simulink model "new_control"  (R2024b)
settings: Solver=FixedStepAuto  StartTime=0.0  StopTime=inf  FixedStep=0.01  RelTol=1e-3  EnableMultiTasking=on
undefined symbols (not defined in the file or in its folder): Discrete, qbreak, Time
libraries: simulink x70, arduinolib x30, dspswit3 x13, arduinosensorlib x2, ctrlSharedLib x2
(part 2 of 4)

== system new_control/Initialize Function/Config_R/Enter Config Mode ==
  Compare To Zero8 : simulink/Logic and Bit Operations/Compare To Zero  relop===  OutDataTypeStr=boolean
  Constant5 : Constant  Value=0x00
  Start_Config_R : arduinolib/I2C Write  I2CModule=0  Mode=Master  SlaveAddress=0x29  SlaveByteOrder=BigEndian  Direction=Transmitter  RegisterAddressMode=on  RegisterAddress=0x3D  SlaveDataType=uint8  DataLength=1  NoAck=off  RepeatedStart=off  OutputStatus=on  blockPlatform=ARDUINO
  Status : Outport
  wires:
  Start_Config_R/1 -> Compare To Zero8/1  "0 for success"
  Constant5/1 -> Start_Config_R/1
  Compare To Zero8/1 -> Status/1

== system new_control/Initialize Function/Config_R/Start Fused (NDOF) Mode ==
  Enable : EnablePort
  Compare To Constant1 : simulink/Logic and Bit Operations/Compare To Constant  relop===  const=0  OutDataTypeStr=boolean
  Constant4 : Constant  Value=0x0C
  I2C Write8 : arduinolib/I2C Write  I2CModule=0  Mode=Master  SlaveAddress=0x29  SlaveByteOrder=BigEndian  Direction=Transmitter  RegisterAddressMode=on  RegisterAddress=0x3D  SlaveDataType=uint8  DataLength=1  NoAck=off  RepeatedStart=off  OutputStatus=on  blockPlatform=ARDUINO
  Status : Outport
  wires:
  Compare To Constant1/1 -> Status/1
  Constant4/1 -> I2C Write8/1
  I2C Write8/1 -> Compare To Constant1/1  "0: success"

== system new_control/Initialize Function/Config_R/X=Z, Y=Y, Z=X ==
  Enable : EnablePort
  Compare To Constant : simulink/Logic and Bit Operations/Compare To Constant  relop=~=  const=hex2dec('06')  OutDataTypeStr=boolean
  Compare To Constant1 : simulink/Logic and Bit Operations/Compare To Constant  relop===  const=hex2dec('06')  OutDataTypeStr=boolean
  Enabled Subsystem : Subsystem  TreatAsAtomicUnit=on
  I2C Read : arduinolib/I2C Read  I2CModule=0  Mode=Master  SlaveAddress=0x29  SlaveByteOrder=LittleEndian  Direction=Receiver  RegisterAddressMode=on  RegisterAddress=0x41  SlaveDataType=uint8  DataLength=1  NoAck=off  RepeatedStart=off  OutputStatus=off  blockPlatform=ARDUINO  SampleTime=-1
  OR : Logic  Operator=OR  IconShape=distinctive  AllPortsSameDT=off  OutDataTypeStr=boolean
  Status : Outport
  wires:
  I2C Read/1 -> Compare To Constant1/1, Compare To Constant/1
  Compare To Constant1/1 -> OR/2
  Compare To Constant/1 -> Enabled Subsystem/Enable
  Enabled Subsystem/1(Status) -> OR/1
  OR/1 -> Status/1

== system new_control/Initialize Function/Config_R/Z = -Z ==
  note: 0x01: Z = -Z
  Enable : EnablePort
  Compare To Constant : simulink/Logic and Bit Operations/Compare To Constant  relop=~=  const=hex2dec('01')  OutDataTypeStr=boolean
  Compare To Constant1 : simulink/Logic and Bit Operations/Compare To Constant  relop===  const=hex2dec('01')  OutDataTypeStr=boolean
  OR : Logic  Operator=OR  IconShape=distinctive  AllPortsSameDT=off  OutDataTypeStr=boolean
  Read : arduinolib/I2C Read  I2CModule=0  Mode=Master  SlaveAddress=0x29  SlaveByteOrder=LittleEndian  Direction=Receiver  RegisterAddressMode=on  RegisterAddress=0x42  SlaveDataType=uint8  DataLength=1  NoAck=off  RepeatedStart=off  OutputStatus=off  blockPlatform=ARDUINO  SampleTime=-1
  Write : Subsystem  TreatAsAtomicUnit=on
  Status : Outport
  wires:
  Write/1(Status) -> OR/1
  Compare To Constant/1 -> Write/Enable
  Read/1 -> Compare To Constant1/1, Compare To Constant/1
  Compare To Constant1/1 -> OR/2
  OR/1 -> Status/1

== system new_control/LEFT LEG/GAIT PHASE BLOCK/CENTERING AND NORMALIZING ==
  Angle max : Inport
  Angle min : Inport  Port=2
  Vel max : Inport  Port=3
  Vel min : Inport  Port=4
  Trigger : TriggerPort  VariantControl=(inherit)  PortDimensions=1
  Abs : Abs  SaturateOnIntegerOverflow=off
  Abs1 : Abs  SaturateOnIntegerOverflow=off
  Constant : Constant  Value=0.5
  Constant1 : Constant  Value=0.5
  Divide : Product  Inputs=/*
  Product : Product
  Product1 : Product
  Sum : Sum
  Sum1 : Sum
  Sum2 : Sum  Inputs=+-
  Sum3 : Sum  Inputs=+-
  Switch : Switch  Criteria=u2 > Threshold  SaturateOnIntegerOverflow=off  InputSameDT=off
  Center vel : Outport
  Center angle : Outport  Port=2
  Gamma : Outport  Port=3
  wires:
  Angle max/1 -> Sum2/1, Sum/1
  Angle min/1 -> Sum2/2, Sum/2
  Sum/1 -> Product/1
  Constant/1 -> Product/2
  Product/1 -> Center angle/1
  Constant1/1 -> Product1/2
  Sum1/1 -> Product1/1
  Vel max/1 -> Sum3/1, Sum1/1
  Vel min/1 -> Sum3/2, Sum1/2
  Product1/1 -> Center vel/1
  Sum2/1 -> Abs/1
  Sum3/1 -> Abs1/1
  Abs/1 -> Switch/2, Switch/1
  Switch/1 -> Divide/1
  Abs1/1 -> Divide/2, Switch/3
  Divide/1 -> Gamma/1

== system new_control/LEFT LEG/GAIT PHASE BLOCK/LOGIC FOR THE BEGINNING ==
  Enable : EnablePort
  Constant : Constant  Value=0
  Phase to zero : Outport
  wires:
  Constant/1 -> Phase to zero/1

== system new_control/LEFT LEG/GAIT PHASE BLOCK/STRIDE EVENT DETECTOR ==
  In1 : Inport
  angle : Inport  Port=2
  Enable : EnablePort
  AND : Logic  IconShape=distinctive  AllPortsSameDT=off  OutDataTypeStr=boolean
  Hit Crossing5 : HitCross  HitCrossingOffset=-0.1  HitCrossingDirection=falling
  Relational Operator : RelationalOperator  OutDataTypeStr=boolean  RndMeth=Simplest  InputSameDT=off
  ~5 degrees : Constant  Value=0.08
  Out1 : Outport
  wires:
  In1/1 -> Hit Crossing5/1
  angle/1 -> Relational Operator/1
  Relational Operator/1 -> AND/2
  ~5 degrees/1 -> Relational Operator/2
  Hit Crossing5/1 -> Out1/1

== system new_control/LEFT LEG/GAIT PHASE BLOCK/Subsystem ==
  Input : Inport
  Trigger : TriggerPort  VariantControl=Variant  PortDimensions=1
  Angle min : Outport
  wires:
  Input/1 -> Angle min/1

== system new_control/LEFT LEG/GAIT PHASE BLOCK/Subsystem2 ==
  Input : Inport
  Trigger : TriggerPort  VariantControl=Variant  PortDimensions=1
  Angle max : Outport
  wires:
  Input/1 -> Angle max/1

== system new_control/LEFT LEG/GAIT PHASE BLOCK/Subsystem4 ==
  Input : Inport
  Trigger : TriggerPort  VariantControl=Variant  PortDimensions=1
  Vel min : Outport
  wires:
  Input/1 -> Vel min/1

== system new_control/LEFT LEG/GAIT PHASE BLOCK/Subsystem5 ==
  Input : Inport
  Trigger : TriggerPort  VariantControl=Variant  PortDimensions=1
  Vel max : Outport
  wires:
  Input/1 -> Vel max/1

== system new_control/LEFT LEG/Subsystem/SIGMOID SCALING ==
  note: a^n / (a^n + 1)
      |
      | The higher n, the more low amplitudes are scaled down
  PORTRAIT RADIUS : Inport
  Sigmoid Power : Inport  Port=2
  Constant2 : Constant
  Divide : Product  Inputs=*/
  Power : Math  Operator=pow
  Scale to 1 : Saturate  UpperLimit=1  LowerLimit=0
  Sum1 : Sum
  Out1 : Outport
  wires:
  Sum1/1 -> Divide/2
  Sigmoid Power/1 -> Power/2  "sig_power_L"
  Constant2/1 -> Sum1/2
  Scale to 1/1 -> Out1/1
  Power/1 -> Divide/1, Sum1/1
  PORTRAIT RADIUS/1 -> Power/1
  Divide/1 -> Scale to 1/1

== system new_control/RIGHT LEG/GAIT PHASE BLOCK/CENTERING AND NORMALIZING ==
  Angle max : Inport
  Angle min : Inport  Port=2
  Vel max : Inport  Port=3
  Vel min : Inport  Port=4
  Trigger : TriggerPort  VariantControl=(inherit)  PortDimensions=1
  Abs : Abs  SaturateOnIntegerOverflow=off
  Abs1 : Abs  SaturateOnIntegerOverflow=off
  Constant : Constant  Value=0.5
  Constant1 : Constant  Value=0.5
  Divide : Product  Inputs=/*
  Product : Product
  Product1 : Product
  Sum : Sum
  Sum1 : Sum
  Sum2 : Sum  Inputs=+-
  Sum3 : Sum  Inputs=+-
  Switch : Switch  Criteria=u2 > Threshold  SaturateOnIntegerOverflow=off  InputSameDT=off
  Center vel : Outport
  Center angle : Outport  Port=2
  Gamma : Outport  Port=3
  wires:
  Angle max/1 -> Sum2/1, Sum/1
  Angle min/1 -> Sum2/2, Sum/2
  Sum/1 -> Product/1
  Constant/1 -> Product/2
  Product/1 -> Center angle/1
  Constant1/1 -> Product1/2
  Sum1/1 -> Product1/1
  Vel max/1 -> Sum3/1, Sum1/1
  Vel min/1 -> Sum3/2, Sum1/2
  Product1/1 -> Center vel/1
  Sum2/1 -> Abs/1
  Sum3/1 -> Abs1/1
  Abs/1 -> Switch/2, Switch/1
  Switch/1 -> Divide/1
  Abs1/1 -> Divide/2, Switch/3
  Divide/1 -> Gamma/1

== system new_control/RIGHT LEG/GAIT PHASE BLOCK/LOGIC FOR THE BEGINNING ==
  Enable : EnablePort
  Constant : Constant  Value=0
  Phase to zero : Outport
  wires:
  Constant/1 -> Phase to zero/1

== system new_control/RIGHT LEG/GAIT PHASE BLOCK/STRIDE EVENT DETECTOR ==
  In1 : Inport
  angle : Inport  Port=2
  Enable : EnablePort
  AND : Logic  IconShape=distinctive  AllPortsSameDT=off  OutDataTypeStr=boolean
  Hit Crossing5 : HitCross  HitCrossingOffset=-0.1  HitCrossingDirection=falling
  Relational Operator : RelationalOperator  OutDataTypeStr=boolean  RndMeth=Simplest  InputSameDT=off
  ~5 degrees : Constant  Value=0.08
  Out1 : Outport
  wires:
  In1/1 -> Hit Crossing5/1
  angle/1 -> Relational Operator/1
  Relational Operator/1 -> AND/2
  ~5 degrees/1 -> Relational Operator/2
  Hit Crossing5/1 -> Out1/1

== system new_control/RIGHT LEG/GAIT PHASE BLOCK/Subsystem ==
  Input : Inport
  Trigger : TriggerPort  VariantControl=Variant  PortDimensions=1
  Angle min : Outport
  wires:
  Input/1 -> Angle min/1

== system new_control/RIGHT LEG/GAIT PHASE BLOCK/Subsystem2 ==
  Input : Inport
  Trigger : TriggerPort  VariantControl=Variant  PortDimensions=1
  Angle max : Outport
  wires:
  Input/1 -> Angle max/1

== system new_control/RIGHT LEG/GAIT PHASE BLOCK/Subsystem4 ==
  Input : Inport
  Trigger : TriggerPort  VariantControl=Variant  PortDimensions=1
  Vel min : Outport
  wires:
  Input/1 -> Vel min/1

== system new_control/RIGHT LEG/GAIT PHASE BLOCK/Subsystem5 ==
  Input : Inport
  Trigger : TriggerPort  VariantControl=Variant  PortDimensions=1
  Vel max : Outport
  wires:
  Input/1 -> Vel max/1

== system new_control/RIGHT LEG/Subsystem/SIGMOID SCALING ==
  note: a^n / (a^n + 1)
      |
      | The higher n, the more low amplitudes are scaled down
  PORTRAIT RADIUS : Inport
  sigmoid_power : Inport  Port=2
  Constant2 : Constant
  Divide : Product  Inputs=*/
  Power : Math  Operator=pow
  Scale to 1 : Saturate  UpperLimit=1  LowerLimit=0
  Sum1 : Sum
  Out1 : Outport
  wires:
  Sum1/1 -> Divide/2
  sigmoid_power/1 -> Power/2
  Constant2/1 -> Sum1/2
  Scale to 1/1 -> Out1/1
  Power/1 -> Divide/1, Sum1/1
  PORTRAIT RADIUS/1 -> Power/1
  Divide/1 -> Scale to 1/1

== system new_control/Subsystem1/Left Motor Velocity1/Motor Actual Position Receive ==
  SWITCH : Inport
  Bus Selector1 : BusSelector  OutputSignals=Data
  CAN Receive : arduinolib/CAN Receive  outputDataType=CAN Msg  identifierType=Standard (11-bit identifier)  messageId=0  msgLength=8  SampleTime=0.01  outputError=off  outputRemote=off
  CHINESE CORRECTION : Subsystem
  Constant1 : Constant  Value=0
  Constant3 : Constant
  Data Type Conversion2 : DataTypeConversion  OutDataTypeStr=uint16  SaturateOnIntegerOverflow=off  RndMeth=Floor
  Delay : Delay  DelayLength=1
  Delay2 : Delay
  Memory2 : Memory
  N-Sample Switch2 : dspswit3/N-Sample Switch  N=10  reset=on  TriggerType=Rising edge  Ts=0.01
  Sum : Sum  Inputs=-|+
  Switch2 : Switch  Criteria=u2 > Threshold  SaturateOnIntegerOverflow=off  InputSameDT=off
  Terminator1 : Terminator
  Unpack2 : Subsystem
  MOTOR POSITION : Outport
  MOTOR SPEED : Outport  Port=2
  MOTOR TORQUE : Outport  Port=3
  wires:
  Switch2/1 -> Sum/1, Delay2/1
  CAN Receive/1 -> Bus Selector1/1
  SWITCH/1 -> N-Sample Switch2/3, CHINESE CORRECTION/Enable
  N-Sample Switch2/1 -> Switch2/2
  Memory2/1 -> Switch2/1
  Constant1/1 -> N-Sample Switch2/1
  Sum/1 -> Delay/1
  Unpack2/2(speed) -> MOTOR SPEED/1  "MOTOR SPEED"
  Delay2/1 -> Memory2/1
  Bus Selector1/1 -> Data Type Conversion2/1  "<Data>"
  CHINESE CORRECTION/1(Out1) -> Sum/2, Switch2/3
  Constant3/1 -> N-Sample Switch2/2
  Unpack2/1(position) -> CHINESE CORRECTION/1(position)  "MOTOR POS"
  Data Type Conversion2/1 -> Unpack2/1(Data)
  CAN Receive/2 -> Terminator1/1
  Delay/1 -> MOTOR POSITION/1
  Unpack2/3(torque) -> MOTOR TORQUE/1  "MOTOR TORQUE"

== system new_control/Subsystem1/Left Motor Velocity1/Subsystem ==
  Motor command : Inport
  SWITCH : Inport  Port=2
  CAN Pack1 : Subsystem
  CAN Transmit1 : arduinolib/CAN Transmit  inputDataType=Raw data  BlockingMode_=on  BlockTimeout_=1  outputStatus=off  identifierType=Standard (11-bit identifier)  messageId=4  msgLength=8  remoteFrame=off
  Constant7 : Constant  Value=0  OutDataTypeStr=single  SampleTime=0.01
  DISABLE1 : Constant  Value=269.7/18  OutDataTypeStr=single
  Data Type Conversion3 : DataTypeConversion  OutDataTypeStr=single  SaturateOnIntegerOverflow=off  RndMeth=Floor
  Demux1 : Demux  Outputs=5
  ENABLE1 : Constant  Value=14.975  OutDataTypeStr=single
  IsNaN : RelationalOperator  Operator=isNaN  OutDataTypeStr=boolean  RndMeth=Simplest  InputSameDT=off
  N-Sample Switch4 : dspswit3/N-Sample Switch  N=15  reset=on  TriggerType=Either edge  Ts=0.01
  Rate Transition : RateTransition  OutPortSampleTime=0.01
  Subsystem2 : Subsystem
  Switch : Switch  Criteria=u2 > Threshold  SaturateOnIntegerOverflow=off  InputSameDT=off
  Switch3 : Switch  Criteria=u2 > Threshold  SaturateOnIntegerOverflow=off  InputSameDT=off
  wires:
  Demux1/4 -> CAN Pack1/4(Kd)
  Data Type Conversion3/1 -> Subsystem2/2(Velocity)
  Switch3/1 -> Subsystem2/1(Enable)
  Demux1/1 -> CAN Pack1/1(Position)
  Motor command/1 -> Data Type Conversion3/1, IsNaN/1
  Demux1/5 -> CAN Pack1/5(Torque)
  ENABLE1/1 -> Switch3/1
  Demux1/2 -> CAN Pack1/2(Velocity)
  Rate Transition/1 -> N-Sample Switch4/3
  IsNaN/1 -> Switch/2
  DISABLE1/1 -> Switch3/3
  Subsystem2/1(Enter_motor_mode) -> N-Sample Switch4/1
  Demux1/3 -> CAN Pack1/3(Kp)
  N-Sample Switch4/1 -> Demux1/1
  Switch/1 -> Rate Transition/1, Switch3/2
  CAN Pack1/1(CAN Data) -> CAN Transmit1/1
  Subsystem2/2(Velocity_value) -> N-Sample Switch4/2
  Constant7/1 -> Switch/1
  SWITCH/1 -> Switch/3

== system new_control/Subsystem1/PID1/Subsystem2 ==
  x : Inport
  Constant : Constant  Value=2
  Integrator1 : Integrator  InitialConditionSource=external
  Integrator2 : Integrator
  Product : Product  RndMeth=Zero
  Product1 : Product  RndMeth=Zero
  Product2 : Product  Inputs=3  RndMeth=Zero
  Sum : Sum  Inputs=|+-
  Sum1 : Sum  Inputs=|+-
  wn : Constant  Value=wn
  x0 : Constant  Value=x0
  zt : Constant  Value=zt
  y : Outport  VectorParamsAs1DForOutWhenUnconnected=off
  yd : Outport  Port=2  VectorParamsAs1DForOutWhenUnconnected=off
  wires:
  Sum/1 -> Product/2
  wn/1 -> Product/1, Product1/1
  Sum1/1 -> Sum/1
  x0/1 -> Integrator1/2
  Integrator2/1 -> Product1/2, Product2/1
  Product/1 -> Integrator2/1
  x/1 -> Sum1/1
  Product1/1 -> Integrator1/1, yd/1
  Integrator1/1 -> Sum1/2, y/1
  Product2/1 -> Sum/2
  zt/1 -> Product2/3
  Constant/1 -> Product2/2

== system new_control/Subsystem1/PID2/Subsystem2 ==
  x : Inport
  Constant : Constant  Value=2
  Integrator1 : Integrator  InitialConditionSource=external
  Integrator2 : Integrator
  Product : Product  RndMeth=Zero
  Product1 : Product  RndMeth=Zero
  Product2 : Product  Inputs=3  RndMeth=Zero
  Sum : Sum  Inputs=|+-
  Sum1 : Sum  Inputs=|+-
  wn : Constant  Value=wn
  x0 : Constant  Value=x0
  zt : Constant  Value=zt
  y : Outport  VectorParamsAs1DForOutWhenUnconnected=off
  yd : Outport  Port=2  VectorParamsAs1DForOutWhenUnconnected=off
  wires:
  Sum/1 -> Product/2
  wn/1 -> Product/1, Product1/1
  Sum1/1 -> Sum/1
  x0/1 -> Integrator1/2
  Integrator2/1 -> Product1/2, Product2/1
  Product/1 -> Integrator2/1
  x/1 -> Sum1/1
  Product1/1 -> Integrator1/1, yd/1
  Integrator1/1 -> Sum1/2, y/1
  Product2/1 -> Sum/2
  zt/1 -> Product2/3
  Constant/1 -> Product2/2

== system new_control/Subsystem1/Right Motor Velocity1/Motor Actual Position Receive ==
  SWITCH : Inport
  Bus Selector1 : BusSelector  OutputSignals=Data
  CAN Receive : arduinolib/CAN Receive  outputDataType=CAN Msg  identifierType=Standard (11-bit identifier)  messageId=0  msgLength=8  SampleTime=0.01  outputError=off  outputRemote=off
  CHINESE CORRECTION : Subsystem
  Constant1 : Constant  Value=0
  Constant3 : Constant
  Data Type Conversion2 : DataTypeConversion  OutDataTypeStr=uint16  SaturateOnIntegerOverflow=off  RndMeth=Floor
  Delay : Delay  DelayLength=1
  Delay2 : Delay
  Memory2 : Memory
  N-Sample Switch2 : dspswit3/N-Sample Switch  N=10  reset=on  TriggerType=Rising edge  Ts=0.01
  Sum : Sum  Inputs=-|+
  Switch2 : Switch  Criteria=u2 > Threshold  SaturateOnIntegerOverflow=off  InputSameDT=off
  Terminator1 : Terminator
  Unpack2 : Subsystem
  MOTOR POSITION : Outport
  MOTOR SPEED : Outport  Port=2
  MOTOR TORQUE : Outport  Port=3
  wires:
  Switch2/1 -> Sum/1, Delay2/1
  CAN Receive/1 -> Bus Selector1/1
  SWITCH/1 -> N-Sample Switch2/3, CHINESE CORRECTION/Enable
  N-Sample Switch2/1 -> Switch2/2
  Memory2/1 -> Switch2/1
  Constant1/1 -> N-Sample Switch2/1
  Sum/1 -> Delay/1
  Unpack2/2(speed) -> MOTOR SPEED/1  "MOTOR SPEED"
  Delay2/1 -> Memory2/1
  Bus Selector1/1 -> Data Type Conversion2/1  "<Data>"
  CHINESE CORRECTION/1(Out1) -> Sum/2, Switch2/3
  Constant3/1 -> N-Sample Switch2/2
  Unpack2/1(position) -> CHINESE CORRECTION/1(position)  "MOTOR POS"
  Data Type Conversion2/1 -> Unpack2/1(Data)
  CAN Receive/2 -> Terminator1/1
  Delay/1 -> MOTOR POSITION/1
  Unpack2/3(torque) -> MOTOR TORQUE/1  "MOTOR TORQUE"

== system new_control/Subsystem1/Right Motor Velocity1/Subsystem ==
  Motor command : Inport
  SWITCH : Inport  Port=2
  CAN Pack1 : Subsystem
  CAN Transmit1 : arduinolib/CAN Transmit  inputDataType=Raw data  BlockingMode_=on  BlockTimeout_=1  outputStatus=off  identifierType=Standard (11-bit identifier)  messageId=3  msgLength=8  remoteFrame=off
  Constant7 : Constant  Value=0  OutDataTypeStr=single  SampleTime=0.01
  DISABLE1 : Constant  Value=269.7/18  OutDataTypeStr=single
  Data Type Conversion3 : DataTypeConversion  OutDataTypeStr=single  SaturateOnIntegerOverflow=off  RndMeth=Floor
  Demux1 : Demux  Outputs=5
  ENABLE1 : Constant  Value=14.975  OutDataTypeStr=single
  IsNaN : RelationalOperator  Operator=isNaN  OutDataTypeStr=boolean  RndMeth=Simplest  InputSameDT=off
  N-Sample Switch4 : dspswit3/N-Sample Switch  N=15  reset=on  TriggerType=Either edge  Ts=0.01
  Rate Transition : RateTransition  OutPortSampleTime=0.01
  Subsystem2 : Subsystem
  Switch : Switch  Criteria=u2 > Threshold  SaturateOnIntegerOverflow=off  InputSameDT=off
  Switch3 : Switch  Criteria=u2 > Threshold  SaturateOnIntegerOverflow=off  InputSameDT=off
  wires:
  Demux1/4 -> CAN Pack1/4(Kd)
  Data Type Conversion3/1 -> Subsystem2/2(Velocity)
  Switch3/1 -> Subsystem2/1(Enable)
  Demux1/1 -> CAN Pack1/1(Position)
  Motor command/1 -> Data Type Conversion3/1, IsNaN/1
  Demux1/5 -> CAN Pack1/5(Torque)
  ENABLE1/1 -> Switch3/1
  Demux1/2 -> CAN Pack1/2(Velocity)
  Rate Transition/1 -> N-Sample Switch4/3
  IsNaN/1 -> Switch/2
  DISABLE1/1 -> Switch3/3
  Subsystem2/1(Enter_motor_mode) -> N-Sample Switch4/1
  Demux1/3 -> CAN Pack1/3(Kp)
  N-Sample Switch4/1 -> Demux1/1
  Switch/1 -> Rate Transition/1, Switch3/2
  CAN Pack1/1(CAN Data) -> CAN Transmit1/1
  Subsystem2/2(Velocity_value) -> N-Sample Switch4/2
  Constant7/1 -> Switch/1
  SWITCH/1 -> Switch/3

== system new_control/Subsystem3/Left Motor Velocity/Motor Actual Position Receive ==
  SWITCH : Inport
  Bus Selector1 : BusSelector  OutputSignals=Data
  CAN Receive : arduinolib/CAN Receive  Priority=4  outputDataType=CAN Msg  identifierType=Standard (11-bit identifier)  messageId=0  msgLength=8  SampleTime=0.01  outputError=off  outputRemote=off
  CHINESE CORRECTION : Subsystem
  Constant1 : Constant  Value=0
  Constant3 : Constant
  Data Type Conversion2 : DataTypeConversion  OutDataTypeStr=uint16  SaturateOnIntegerOverflow=off  RndMeth=Floor
  Delay : Delay  DelayLength=1
  Delay2 : Delay
  Memory2 : Memory
  N-Sample Switch2 : dspswit3/N-Sample Switch  N=10  reset=on  TriggerType=Rising edge  Ts=0.01
  Sum : Sum  Inputs=-|+
  Switch2 : Switch  Criteria=u2 > Threshold  SaturateOnIntegerOverflow=off  InputSameDT=off
  Terminator1 : Terminator
  Unpack2 : Subsystem
  Zero-Order Hold1 : ZeroOrderHold  SampleTime=0.01
  MOTOR POSITION : Outport
  MOTOR SPEED : Outport  Port=2
  MOTOR TORQUE : Outport  Port=3
  wires:
  Switch2/1 -> Sum/1, Delay2/1
  CAN Receive/1 -> Bus Selector1/1
  SWITCH/1 -> Zero-Order Hold1/1
  N-Sample Switch2/1 -> Switch2/2
  Memory2/1 -> Switch2/1
  Constant1/1 -> N-Sample Switch2/1
  Sum/1 -> Delay/1
  Unpack2/2(speed) -> MOTOR SPEED/1  "MOTOR SPEED"
  Delay2/1 -> Memory2/1
  Bus Selector1/1 -> Data Type Conversion2/1  "<Data>"
  CHINESE CORRECTION/1(Out1) -> Sum/2, Switch2/3
  Constant3/1 -> N-Sample Switch2/2
  Unpack2/1(position) -> CHINESE CORRECTION/1(position)  "MOTOR POS"
  Data Type Conversion2/1 -> Unpack2/1(Data)
  CAN Receive/2 -> Terminator1/1
  Delay/1 -> MOTOR POSITION/1
  Unpack2/3(torque) -> MOTOR TORQUE/1  "MOTOR TORQUE"
  Zero-Order Hold1/1 -> N-Sample Switch2/3, CHINESE CORRECTION/Enable

== system new_control/Subsystem3/Left Motor Velocity/Subsystem ==
  Motor command : Inport
  SWITCH : Inport  Port=2
  CAN Pack1 : Subsystem
  CAN Transmit1 : arduinolib/CAN Transmit  Priority=3  inputDataType=Raw data  BlockingMode_=on  BlockTimeout_=1  outputStatus=off  identifierType=Standard (11-bit identifier)  messageId=4  msgLength=8  remoteFrame=off
  Constant7 : Constant  Value=0  OutDataTypeStr=single  SampleTime=0.01
  DISABLE1 : Constant  Value=269.7/18  OutDataTypeStr=single
  Data Type Conversion3 : DataTypeConversion  OutDataTypeStr=single  SaturateOnIntegerOverflow=off  RndMeth=Floor
  Demux1 : Demux  Outputs=5
  ENABLE1 : Constant  Value=14.975  OutDataTypeStr=single
  IsNaN : RelationalOperator  Operator=isNaN  OutDataTypeStr=boolean  RndMeth=Simplest  InputSameDT=off
  N-Sample Switch4 : dspswit3/N-Sample Switch  N=15  reset=on  TriggerType=Either edge  Ts=0.01
  Rate Transition : RateTransition  OutPortSampleTime=0.01
  Subsystem2 : Subsystem
  Switch : Switch  Criteria=u2 > Threshold  SaturateOnIntegerOverflow=off  InputSameDT=off
  Switch3 : Switch  Criteria=u2 > Threshold  SaturateOnIntegerOverflow=off  InputSameDT=off
  wires:
  Demux1/4 -> CAN Pack1/4(Kd)
  Data Type Conversion3/1 -> Subsystem2/2(Velocity)
  Switch3/1 -> Subsystem2/1(Enable)
  Demux1/1 -> CAN Pack1/1(Position)
  Motor command/1 -> Data Type Conversion3/1, IsNaN/1
  Demux1/5 -> CAN Pack1/5(Torque)
  ENABLE1/1 -> Switch3/1
  Demux1/2 -> CAN Pack1/2(Velocity)
  Rate Transition/1 -> N-Sample Switch4/3
  IsNaN/1 -> Switch/2
  DISABLE1/1 -> Switch3/3
  Subsystem2/1(Enter_motor_mode) -> N-Sample Switch4/1
  Demux1/3 -> CAN Pack1/3(Kp)
  N-Sample Switch4/1 -> Demux1/1
  Switch/1 -> Rate Transition/1, Switch3/2
  CAN Pack1/1(CAN Data) -> CAN Transmit1/1
  Subsystem2/2(Velocity_value) -> N-Sample Switch4/2
  Constant7/1 -> Switch/1
  SWITCH/1 -> Switch/3

== system new_control/Subsystem3/Right Motor Velocity/Motor Actual Position Receive ==
  SWITCH : Inport
  Bus Selector1 : BusSelector  OutputSignals=Data
  CAN Receive : arduinolib/CAN Receive  Priority=2  outputDataType=CAN Msg  identifierType=Standard (11-bit identifier)  messageId=0  msgLength=8  SampleTime=0.01  outputError=off  outputRemote=off
  CHINESE CORRECTION : Subsystem
  Constant1 : Constant  Value=0
  Constant3 : Constant
  Data Type Conversion2 : DataTypeConversion  OutDataTypeStr=uint16  SaturateOnIntegerOverflow=off  RndMeth=Floor
  Delay : Delay  DelayLength=1
  Delay2 : Delay
  Memory2 : Memory
  N-Sample Switch2 : dspswit3/N-Sample Switch  N=10  reset=on  TriggerType=Rising edge  Ts=0.01
  Sum : Sum  Inputs=-|+
  Switch2 : Switch  Criteria=u2 > Threshold  SaturateOnIntegerOverflow=off  InputSameDT=off
  Terminator1 : Terminator
  Unpack2 : Subsystem
  Zero-Order Hold1 : ZeroOrderHold  SampleTime=0.01
  MOTOR POSITION : Outport
  MOTOR SPEED : Outport  Port=2
  MOTOR TORQUE : Outport  Port=3
  wires:
  Switch2/1 -> Sum/1, Delay2/1
  CAN Receive/1 -> Bus Selector1/1
  SWITCH/1 -> Zero-Order Hold1/1
  N-Sample Switch2/1 -> Switch2/2
  Memory2/1 -> Switch2/1
  Constant1/1 -> N-Sample Switch2/1
  Sum/1 -> Delay/1
  Unpack2/2(speed) -> MOTOR SPEED/1  "MOTOR SPEED"
  Delay2/1 -> Memory2/1
  Bus Selector1/1 -> Data Type Conversion2/1  "<Data>"
  CHINESE CORRECTION/1(Out1) -> Sum/2, Switch2/3
  Constant3/1 -> N-Sample Switch2/2
  Unpack2/1(position) -> CHINESE CORRECTION/1(position)  "MOTOR POS"
  Data Type Conversion2/1 -> Unpack2/1(Data)
  CAN Receive/2 -> Terminator1/1
  Delay/1 -> MOTOR POSITION/1
  Unpack2/3(torque) -> MOTOR TORQUE/1  "MOTOR TORQUE"
  Zero-Order Hold1/1 -> N-Sample Switch2/3, CHINESE CORRECTION/Enable

== system new_control/Subsystem3/Right Motor Velocity/Subsystem ==
  Motor command : Inport
  SWITCH : Inport  Port=2
  CAN Pack1 : Subsystem
  CAN Transmit1 : arduinolib/CAN Transmit  Priority=1  inputDataType=Raw data  BlockingMode_=on  BlockTimeout_=1  outputStatus=off  identifierType=Standard (11-bit identifier)  messageId=3  msgLength=8  remoteFrame=off
  Constant7 : Constant  Value=0  OutDataTypeStr=single  SampleTime=0.01
  DISABLE1 : Constant  Value=269.7/18  OutDataTypeStr=single
  Data Type Conversion3 : DataTypeConversion  OutDataTypeStr=single  SaturateOnIntegerOverflow=off  RndMeth=Floor
  Demux1 : Demux  Outputs=5
  ENABLE1 : Constant  Value=14.975  OutDataTypeStr=single
  IsNaN : RelationalOperator  Operator=isNaN  OutDataTypeStr=boolean  RndMeth=Simplest  InputSameDT=off
  N-Sample Switch4 : dspswit3/N-Sample Switch  N=15  reset=on  TriggerType=Either edge  Ts=0.01
  Rate Transition : RateTransition  OutPortSampleTime=0.01
  Subsystem2 : Subsystem
  Switch : Switch  Criteria=u2 > Threshold  SaturateOnIntegerOverflow=off  InputSameDT=off
  Switch3 : Switch  Criteria=u2 > Threshold  SaturateOnIntegerOverflow=off  InputSameDT=off
  wires:
  Demux1/4 -> CAN Pack1/4(Kd)
  Data Type Conversion3/1 -> Subsystem2/2(Velocity)
  Switch3/1 -> Subsystem2/1(Enable)
  Demux1/1 -> CAN Pack1/1(Position)
  Motor command/1 -> Data Type Conversion3/1, IsNaN/1
  Demux1/5 -> CAN Pack1/5(Torque)
  ENABLE1/1 -> Switch3/1
  Demux1/2 -> CAN Pack1/2(Velocity)
  Rate Transition/1 -> N-Sample Switch4/3
  IsNaN/1 -> Switch/2
  DISABLE1/1 -> Switch3/3
  Subsystem2/1(Enter_motor_mode) -> N-Sample Switch4/1
  Demux1/3 -> CAN Pack1/3(Kp)
  N-Sample Switch4/1 -> Demux1/1
  Switch/1 -> Rate Transition/1, Switch3/2
  CAN Pack1/1(CAN Data) -> CAN Transmit1/1
  Subsystem2/2(Velocity_value) -> N-Sample Switch4/2
  Constant7/1 -> Switch/1
  SWITCH/1 -> Switch/3

== system new_control/Initialize Function/Config_L /X=Z, Y=Y, Z=X/Enabled Subsystem ==
  Enable : EnablePort
  Compare To Constant1 : simulink/Logic and Bit Operations/Compare To Constant  relop===  const=0  OutDataTypeStr=boolean
  Constant2 : Constant  Value=0x06
  I2C Write6 : arduinolib/I2C Write  I2CModule=0  Mode=Master  SlaveAddress=0x28  SlaveByteOrder=BigEndian  Direction=Transmitter  RegisterAddressMode=on  RegisterAddress=0x41  SlaveDataType=uint8  DataLength=1  NoAck=off  RepeatedStart=off  OutputStatus=on  blockPlatform=ARDUINO
  Status : Outport
  wires:
  Constant2/1 -> I2C Write6/1
  I2C Write6/1 -> Compare To Constant1/1  "0: success"
  Compare To Constant1/1 -> Status/1

== system new_control/Initialize Function/Config_L /Z = -Z/Write ==
  Enable : EnablePort
  Compare To Constant1 : simulink/Logic and Bit Operations/Compare To Constant  relop===  const=0  OutDataTypeStr=boolean
  Constant2 : Constant  Value=0x01
  I2C Write7 : arduinolib/I2C Write  I2CModule=0  Mode=Master  SlaveAddress=0x28  SlaveByteOrder=BigEndian  Direction=Transmitter  RegisterAddressMode=on  RegisterAddress=0x42  SlaveDataType=uint8  DataLength=1  NoAck=off  RepeatedStart=off  OutputStatus=on  blockPlatform=ARDUINO
  Status : Outport
  wires:
  Constant2/1 -> I2C Write7/1
  I2C Write7/1 -> Compare To Constant1/1  "0: success"
  Compare To Constant1/1 -> Status/1

== system new_control/Initialize Function/Config_R/X=Z, Y=Y, Z=X/Enabled Subsystem ==
  Enable : EnablePort
  Compare To Constant1 : simulink/Logic and Bit Operations/Compare To Constant  relop===  const=0  OutDataTypeStr=boolean
  Constant2 : Constant  Value=0x06
  I2C Write6 : arduinolib/I2C Write  I2CModule=0  Mode=Master  SlaveAddress=0x29  SlaveByteOrder=BigEndian  Direction=Transmitter  RegisterAddressMode=on  RegisterAddress=0x41  SlaveDataType=uint8  DataLength=1  NoAck=off  RepeatedStart=off  OutputStatus=on  blockPlatform=ARDUINO
  Status : Outport
  wires:
  Constant2/1 -> I2C Write6/1
  I2C Write6/1 -> Compare To Constant1/1  "0: success"
  Compare To Constant1/1 -> Status/1

== system new_control/Initialize Function/Config_R/Z = -Z/Write ==
  Enable : EnablePort
  Compare To Constant1 : simulink/Logic and Bit Operations/Compare To Constant  relop===  const=0  OutDataTypeStr=boolean
  Constant2 : Constant  Value=0x01
  I2C Write7 : arduinolib/I2C Write  I2CModule=0  Mode=Master  SlaveAddress=0x29  SlaveByteOrder=BigEndian  Direction=Transmitter  RegisterAddressMode=on  RegisterAddress=0x42  SlaveDataType=uint8  DataLength=1  NoAck=off  RepeatedStart=off  OutputStatus=on  blockPlatform=ARDUINO
  Status : Outport
  wires:
  Constant2/1 -> I2C Write7/1
  I2C Write7/1 -> Compare To Constant1/1  "0: success"
  Compare To Constant1/1 -> Status/1

== system new_control/Subsystem1/Left Motor Velocity1/Motor Actual Position Receive/CHINESE CORRECTION ==
  position : Inport
  Enable : EnablePort  StatesWhenEnabling=reset
  Abs : Abs  SaturateOnIntegerOverflow=off
  Constant2 : Constant
  Constant3 : Constant  Value=0
  Memory : Memory
  Subsystem : Subsystem
  Sum : Sum  Inputs=|+-
  Sum1 : Sum  Inputs=+-
  Switch1 : Switch  Criteria=u2 > Threshold  Threshold=20  SaturateOnIntegerOverflow=off  InputSameDT=off
  Out1 : Outport
  wires:
  Constant2/1 -> Switch1/1
  position/1 -> Sum1/1, Sum/1, Memory/1
  Sum/1 -> Abs/1, Subsystem/1(In1)
  Sum1/1 -> Out1/1
  Abs/1 -> Switch1/2
  Constant3/1 -> Switch1/3
  Switch1/1 -> Subsystem/Enable
  Memory/1 -> Sum/2
  Subsystem/1(Out1) -> Sum1/2

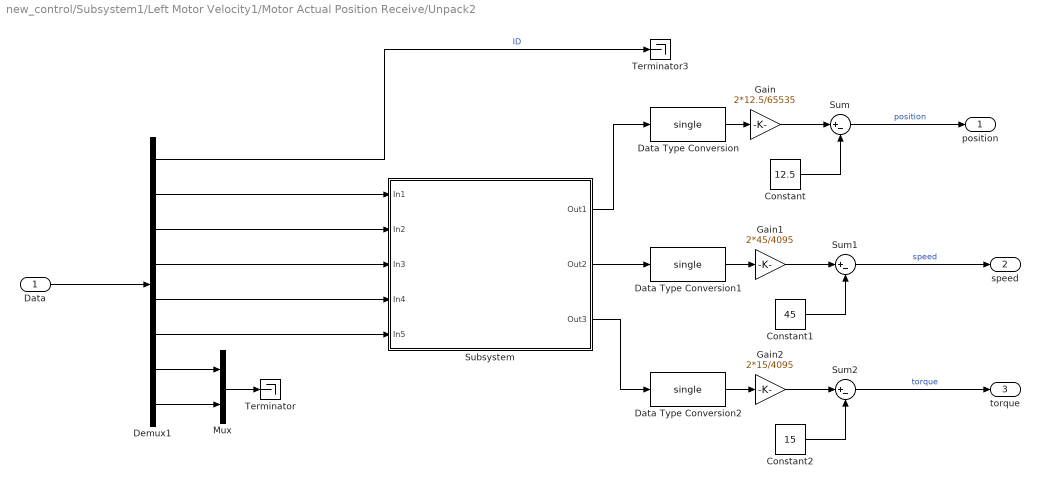
== system new_control/Subsystem1/Left Motor Velocity1/Motor Actual Position Receive/Unpack2 ==
  Data : Inport
  Constant : Constant  Value=12.5
  Constant1 : Constant  Value=45
  Constant2 : Constant  Value=15
  Data Type Conversion : DataTypeConversion  OutDataTypeStr=single  SaturateOnIntegerOverflow=off  RndMeth=Floor
  Data Type Conversion1 : DataTypeConversion  OutDataTypeStr=single  SaturateOnIntegerOverflow=off  RndMeth=Floor
  Data Type Conversion2 : DataTypeConversion  OutDataTypeStr=single  SaturateOnIntegerOverflow=off  RndMeth=Floor
  Demux1 : Demux  Outputs=8
  Gain : Gain  Gain=2*12.5/65535  RndMeth=Round
  Gain1 : Gain  Gain=2*45/4095  RndMeth=Round
  Gain2 : Gain  Gain=2*15/4095  RndMeth=Round
  Mux : Mux  Inputs=2
  Subsystem : Subsystem
  Sum : Sum  Inputs=|+-
  Sum1 : Sum  Inputs=|+-
  Sum2 : Sum  Inputs=|+-
  Terminator : Terminator
  Terminator3 : Terminator
  position : Outport
  speed : Outport  Port=2
  torque : Outport  Port=3
  wires:
  Demux1/1 -> Terminator3/1  "ID"
  Demux1/7 -> Mux/1
  Demux1/8 -> Mux/2
  Demux1/2 -> Subsystem/1(In1)
  Demux1/3 -> Subsystem/2(In2)
  Demux1/4 -> Subsystem/3(In3)
  Demux1/5 -> Subsystem/4(In4)
  Demux1/6 -> Subsystem/5(In5)
  Subsystem/1(Out1) -> Data Type Conversion/1
  Gain/1 -> Sum/1
  Constant/1 -> Sum/2
  Data Type Conversion/1 -> Gain/1
  Gain1/1 -> Sum1/1
  Data Type Conversion1/1 -> Gain1/1
  Constant1/1 -> Sum1/2
  Gain2/1 -> Sum2/1
  Data Type Conversion2/1 -> Gain2/1
  Constant2/1 -> Sum2/2
  Subsystem/2(Out2) -> Data Type Conversion1/1
  Subsystem/3(Out3) -> Data Type Conversion2/1
  Sum2/1 -> torque/1  "torque"
  Mux/1 -> Terminator/1
  Data/1 -> Demux1/1
  Sum/1 -> position/1  "position"
  Sum1/1 -> speed/1  "speed"

== system new_control/Subsystem1/Left Motor Velocity1/Subsystem/CAN Pack1 ==
  Position : Inport
  Velocity : Inport  Port=2
  Kp : Inport  Port=3
  Kd : Inport  Port=4
  Torque : Inport  Port=5
  Constant3 : Constant  Value=-12.5  OutDataTypeStr=single
  Constant4 : Constant  Value=-45  OutDataTypeStr=single
  Constant5 : Constant  Value=-15  OutDataTypeStr=single
  Gain : Gain  Gain=65535/(2*12.5)  OutDataTypeStr=uint16  RndMeth=Round
  Gain3 : Gain  Gain=4095/(2*45)  OutDataTypeStr=fixdt(0,12,0)  RndMeth=Round
  Gain4 : Gain  Gain=4095/500  OutDataTypeStr=fixdt(0,12,0)  RndMeth=Round
  Gain5 : Gain  Gain=4095/5  OutDataTypeStr=fixdt(0,12,0)  RndMeth=Round
  Gain6 : Gain  Gain=4095/(2*15)  OutDataTypeStr=fixdt(0,12,0)  RndMeth=Round
  Subsystem : Subsystem
  Sum3 : Sum  Inputs=|+-
  Sum4 : Sum  Inputs=|+-
  Sum5 : Sum  Inputs=|+-
  Vector Concatenate : Concatenate  NumInputs=8
  CAN Data : Outport
  wires:
  Velocity/1 -> Sum4/1
  Kp/1 -> Gain4/1
  Kd/1 -> Gain5/1
  Vector Concatenate/1 -> CAN Data/1
  Constant3/1 -> Sum3/2
  Sum3/1 -> Gain/1  "position"
  Position/1 -> Sum3/1
  Constant4/1 -> Sum4/2
  Constant5/1 -> Sum5/2
  Sum5/1 -> Gain6/1  "torque"
  Torque/1 -> Sum5/1
  Sum4/1 -> Gain3/1  "speed"
  Gain/1 -> Subsystem/1(p_int)
  Gain3/1 -> Subsystem/2(v_int)
  Gain4/1 -> Subsystem/3(kp_int)
  Gain5/1 -> Subsystem/4(kd_int)
  Gain6/1 -> Subsystem/5(t_int)
  Subsystem/1(Out2) -> Vector Concatenate/1
  Subsystem/2(Out1) -> Vector Concatenate/2
  Subsystem/4(Out4) -> Vector Concatenate/4
  Subsystem/5(Out5) -> Vector Concatenate/5
  Subsystem/6(Out6) -> Vector Concatenate/6
  Subsystem/7(Out7) -> Vector Concatenate/7
  Subsystem/3(Out3) -> Vector Concatenate/3
  Subsystem/8(Out8) -> Vector Concatenate/8

== system new_control/Subsystem1/Left Motor Velocity1/Subsystem/Subsystem2 ==
  Enable : Inport
  Velocity : Inport  Port=2
  Mux1 : Mux  Inputs=5
  Subsystem : Subsystem
  Subsystem2 : Subsystem
  Enter_motor_mode : Outport
  Velocity_value : Outport  Port=2
  wires:
  Subsystem2/3(Out3) -> Mux1/3
  Subsystem2/2(Out2) -> Mux1/2
  Subsystem2/4(Out4) -> Mux1/4
  Subsystem2/1(Out1) -> Mux1/1
  Subsystem/1(Out1) -> Velocity_value/1
  Mux1/1 -> Enter_motor_mode/1
  Enable/1 -> Mux1/5
  Velocity/1 -> Subsystem/1(In1)

== system new_control/Subsystem1/Right Motor Velocity1/Motor Actual Position Receive/CHINESE CORRECTION ==
  position : Inport
  Enable : EnablePort  StatesWhenEnabling=reset
  Abs : Abs  SaturateOnIntegerOverflow=off
  Constant2 : Constant
  Constant3 : Constant  Value=0
  Memory : Memory
  Subsystem : Subsystem
  Sum : Sum  Inputs=|+-
  Sum1 : Sum  Inputs=+-
  Switch1 : Switch  Criteria=u2 > Threshold  Threshold=20  SaturateOnIntegerOverflow=off  InputSameDT=off
  Out1 : Outport
  wires:
  Constant2/1 -> Switch1/1
  position/1 -> Sum1/1, Sum/1, Memory/1
  Sum/1 -> Abs/1, Subsystem/1(In1)
  Sum1/1 -> Out1/1
  Abs/1 -> Switch1/2
  Constant3/1 -> Switch1/3
  Switch1/1 -> Subsystem/Enable
  Memory/1 -> Sum/2
  Subsystem/1(Out1) -> Sum1/2

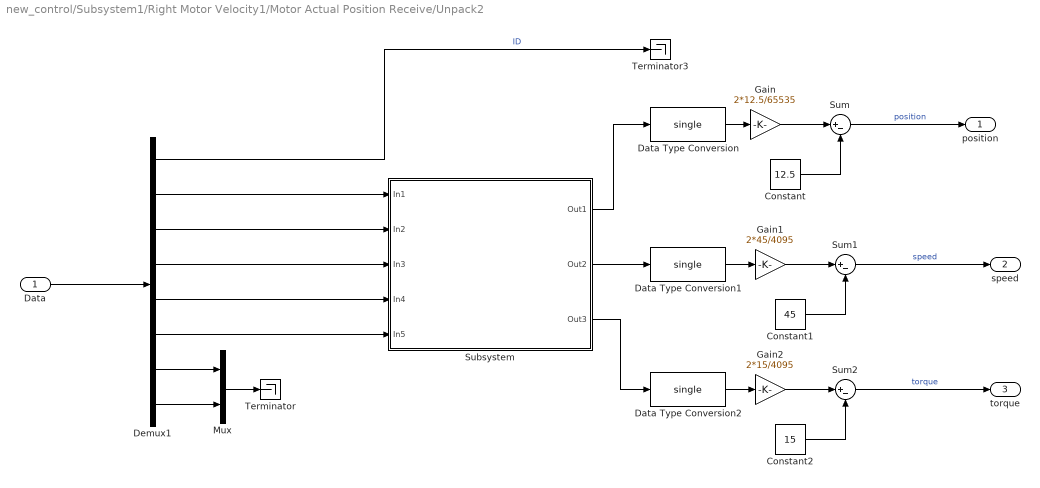
== system new_control/Subsystem1/Right Motor Velocity1/Motor Actual Position Receive/Unpack2 ==
  Data : Inport
  Constant : Constant  Value=12.5
  Constant1 : Constant  Value=45
  Constant2 : Constant  Value=15
  Data Type Conversion : DataTypeConversion  OutDataTypeStr=single  SaturateOnIntegerOverflow=off  RndMeth=Floor
  Data Type Conversion1 : DataTypeConversion  OutDataTypeStr=single  SaturateOnIntegerOverflow=off  RndMeth=Floor
  Data Type Conversion2 : DataTypeConversion  OutDataTypeStr=single  SaturateOnIntegerOverflow=off  RndMeth=Floor
  Demux1 : Demux  Outputs=8
  Gain : Gain  Gain=2*12.5/65535  RndMeth=Round
  Gain1 : Gain  Gain=2*45/4095  RndMeth=Round
  Gain2 : Gain  Gain=2*15/4095  RndMeth=Round
  Mux : Mux  Inputs=2
  Subsystem : Subsystem
  Sum : Sum  Inputs=|+-
  Sum1 : Sum  Inputs=|+-
  Sum2 : Sum  Inputs=|+-
  Terminator : Terminator
  Terminator3 : Terminator
  position : Outport
  speed : Outport  Port=2
  torque : Outport  Port=3
  wires:
  Demux1/1 -> Terminator3/1  "ID"
  Demux1/7 -> Mux/1
  Demux1/8 -> Mux/2
  Demux1/2 -> Subsystem/1(In1)
  Demux1/3 -> Subsystem/2(In2)
  Demux1/4 -> Subsystem/3(In3)
  Demux1/5 -> Subsystem/4(In4)
  Demux1/6 -> Subsystem/5(In5)
  Subsystem/1(Out1) -> Data Type Conversion/1
  Gain/1 -> Sum/1
  Constant/1 -> Sum/2
  Data Type Conversion/1 -> Gain/1
  Gain1/1 -> Sum1/1
  Data Type Conversion1/1 -> Gain1/1
  Constant1/1 -> Sum1/2
  Gain2/1 -> Sum2/1
  Data Type Conversion2/1 -> Gain2/1
  Constant2/1 -> Sum2/2
  Subsystem/2(Out2) -> Data Type Conversion1/1
  Subsystem/3(Out3) -> Data Type Conversion2/1
  Sum2/1 -> torque/1  "torque"
  Mux/1 -> Terminator/1
  Data/1 -> Demux1/1
  Sum/1 -> position/1  "position"
  Sum1/1 -> speed/1  "speed"

== system new_control/Subsystem1/Right Motor Velocity1/Subsystem/CAN Pack1 ==
  Position : Inport
  Velocity : Inport  Port=2
  Kp : Inport  Port=3
  Kd : Inport  Port=4
  Torque : Inport  Port=5
  Constant3 : Constant  Value=-12.5  OutDataTypeStr=single
  Constant4 : Constant  Value=-45  OutDataTypeStr=single
  Constant5 : Constant  Value=-15  OutDataTypeStr=single
  Gain : Gain  Gain=65535/(2*12.5)  OutDataTypeStr=uint16  RndMeth=Round
  Gain3 : Gain  Gain=4095/(2*45)  OutDataTypeStr=fixdt(0,12,0)  RndMeth=Round
  Gain4 : Gain  Gain=4095/500  OutDataTypeStr=fixdt(0,12,0)  RndMeth=Round
  Gain5 : Gain  Gain=4095/5  OutDataTypeStr=fixdt(0,12,0)  RndMeth=Round
  Gain6 : Gain  Gain=4095/(2*15)  OutDataTypeStr=fixdt(0,12,0)  RndMeth=Round
  Subsystem : Subsystem
  Sum3 : Sum  Inputs=|+-
  Sum4 : Sum  Inputs=|+-
  Sum5 : Sum  Inputs=|+-
  Vector Concatenate : Concatenate  NumInputs=8
  CAN Data : Outport
  wires:
  Velocity/1 -> Sum4/1
  Kp/1 -> Gain4/1
  Kd/1 -> Gain5/1
  Vector Concatenate/1 -> CAN Data/1
  Constant3/1 -> Sum3/2
  Sum3/1 -> Gain/1  "position"
  Position/1 -> Sum3/1
  Constant4/1 -> Sum4/2
  Constant5/1 -> Sum5/2
  Sum5/1 -> Gain6/1  "torque"
  Torque/1 -> Sum5/1
  Sum4/1 -> Gain3/1  "speed"
  Gain/1 -> Subsystem/1(p_int)
  Gain3/1 -> Subsystem/2(v_int)
  Gain4/1 -> Subsystem/3(kp_int)
  Gain5/1 -> Subsystem/4(kd_int)
  Gain6/1 -> Subsystem/5(t_int)
  Subsystem/1(Out2) -> Vector Concatenate/1
  Subsystem/2(Out1) -> Vector Concatenate/2
  Subsystem/4(Out4) -> Vector Concatenate/4
  Subsystem/5(Out5) -> Vector Concatenate/5
  Subsystem/6(Out6) -> Vector Concatenate/6
  Subsystem/7(Out7) -> Vector Concatenate/7
  Subsystem/3(Out3) -> Vector Concatenate/3
  Subsystem/8(Out8) -> Vector Concatenate/8

== system new_control/Subsystem1/Right Motor Velocity1/Subsystem/Subsystem2 ==
  Enable : Inport
  Velocity : Inport  Port=2
  Mux1 : Mux  Inputs=5
  Subsystem : Subsystem
  Subsystem2 : Subsystem
  Enter_motor_mode : Outport
  Velocity_value : Outport  Port=2
  wires:
  Subsystem2/3(Out3) -> Mux1/3
  Subsystem2/2(Out2) -> Mux1/2
  Subsystem2/4(Out4) -> Mux1/4
  Subsystem2/1(Out1) -> Mux1/1
  Subsystem/1(Out1) -> Velocity_value/1
  Mux1/1 -> Enter_motor_mode/1
  Enable/1 -> Mux1/5
  Velocity/1 -> Subsystem/1(In1)

== system new_control/Subsystem3/Left Motor Velocity/Motor Actual Position Receive/CHINESE CORRECTION ==
  position : Inport
  Enable : EnablePort  StatesWhenEnabling=reset
  Abs : Abs  SaturateOnIntegerOverflow=off
  Constant2 : Constant
  Constant3 : Constant  Value=0
  Memory : Memory
  Subsystem : Subsystem
  Sum : Sum  Inputs=|+-
  Sum1 : Sum  Inputs=+-
  Switch1 : Switch  Criteria=u2 > Threshold  Threshold=20  SaturateOnIntegerOverflow=off  InputSameDT=off
  Out1 : Outport
  wires:
  Constant2/1 -> Switch1/1
  position/1 -> Sum1/1, Sum/1, Memory/1
  Sum/1 -> Abs/1, Subsystem/1(In1)
  Sum1/1 -> Out1/1
  Abs/1 -> Switch1/2
  Constant3/1 -> Switch1/3
  Switch1/1 -> Subsystem/Enable
  Memory/1 -> Sum/2
  Subsystem/1(Out1) -> Sum1/2

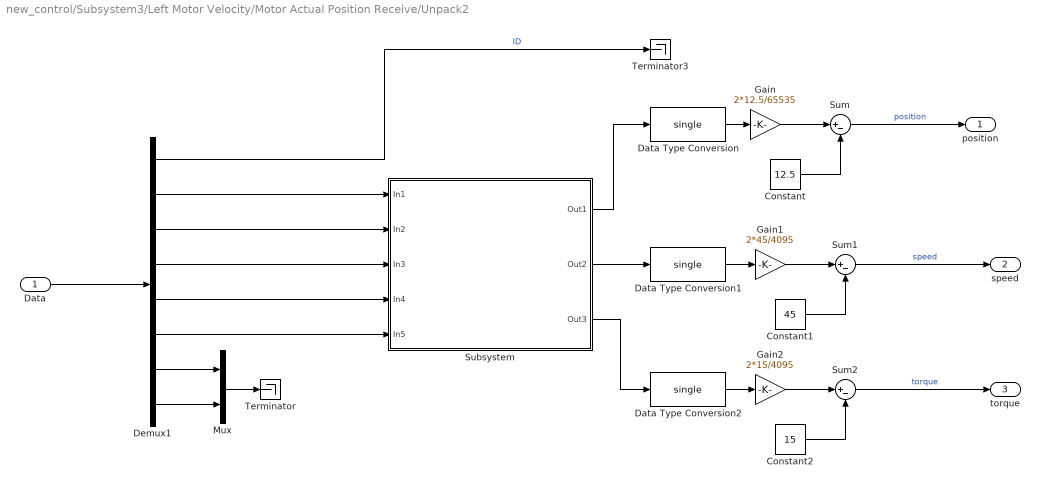
== system new_control/Subsystem3/Left Motor Velocity/Motor Actual Position Receive/Unpack2 ==
  Data : Inport
  Constant : Constant  Value=12.5
  Constant1 : Constant  Value=45
  Constant2 : Constant  Value=15
  Data Type Conversion : DataTypeConversion  OutDataTypeStr=single  SaturateOnIntegerOverflow=off  RndMeth=Floor
  Data Type Conversion1 : DataTypeConversion  OutDataTypeStr=single  SaturateOnIntegerOverflow=off  RndMeth=Floor
  Data Type Conversion2 : DataTypeConversion  OutDataTypeStr=single  SaturateOnIntegerOverflow=off  RndMeth=Floor
  Demux1 : Demux  Outputs=8
  Gain : Gain  Gain=2*12.5/65535  RndMeth=Round
  Gain1 : Gain  Gain=2*45/4095  RndMeth=Round
  Gain2 : Gain  Gain=2*15/4095  RndMeth=Round
  Mux : Mux  Inputs=2
  Subsystem : Subsystem
  Sum : Sum  Inputs=|+-
  Sum1 : Sum  Inputs=|+-
  Sum2 : Sum  Inputs=|+-
  Terminator : Terminator
  Terminator3 : Terminator
  position : Outport
  speed : Outport  Port=2
  torque : Outport  Port=3
  wires:
  Demux1/1 -> Terminator3/1  "ID"
  Demux1/7 -> Mux/1
  Demux1/8 -> Mux/2
  Demux1/2 -> Subsystem/1(In1)
  Demux1/3 -> Subsystem/2(In2)
  Demux1/4 -> Subsystem/3(In3)
  Demux1/5 -> Subsystem/4(In4)
  Demux1/6 -> Subsystem/5(In5)
  Subsystem/1(Out1) -> Data Type Conversion/1
  Gain/1 -> Sum/1
  Constant/1 -> Sum/2
  Data Type Conversion/1 -> Gain/1
  Gain1/1 -> Sum1/1
  Data Type Conversion1/1 -> Gain1/1
  Constant1/1 -> Sum1/2
  Gain2/1 -> Sum2/1
  Data Type Conversion2/1 -> Gain2/1
  Constant2/1 -> Sum2/2
  Subsystem/2(Out2) -> Data Type Conversion1/1
  Subsystem/3(Out3) -> Data Type Conversion2/1
  Sum2/1 -> torque/1  "torque"
  Mux/1 -> Terminator/1
  Data/1 -> Demux1/1
  Sum/1 -> position/1  "position"
  Sum1/1 -> speed/1  "speed"

== system new_control/Subsystem3/Left Motor Velocity/Subsystem/CAN Pack1 ==
  Position : Inport
  Velocity : Inport  Port=2
  Kp : Inport  Port=3
  Kd : Inport  Port=4
  Torque : Inport  Port=5
  Constant3 : Constant  Value=-12.5  OutDataTypeStr=single
  Constant4 : Constant  Value=-45  OutDataTypeStr=single
  Constant5 : Constant  Value=-15  OutDataTypeStr=single
  Gain : Gain  Gain=65535/(2*12.5)  OutDataTypeStr=uint16  RndMeth=Round
  Gain3 : Gain  Gain=4095/(2*45)  OutDataTypeStr=fixdt(0,12,0)  RndMeth=Round
  Gain4 : Gain  Gain=4095/500  OutDataTypeStr=fixdt(0,12,0)  RndMeth=Round
  Gain5 : Gain  Gain=4095/5  OutDataTypeStr=fixdt(0,12,0)  RndMeth=Round
  Gain6 : Gain  Gain=4095/(2*15)  OutDataTypeStr=fixdt(0,12,0)  RndMeth=Round
  Subsystem : Subsystem
  Sum3 : Sum  Inputs=|+-
  Sum4 : Sum  Inputs=|+-
  Sum5 : Sum  Inputs=|+-
  Vector Concatenate : Concatenate  NumInputs=8
  CAN Data : Outport
  wires:
  Velocity/1 -> Sum4/1
  Kp/1 -> Gain4/1
  Kd/1 -> Gain5/1
  Vector Concatenate/1 -> CAN Data/1
  Constant3/1 -> Sum3/2
  Sum3/1 -> Gain/1  "position"
  Position/1 -> Sum3/1
  Constant4/1 -> Sum4/2
  Constant5/1 -> Sum5/2
  Sum5/1 -> Gain6/1  "torque"
  Torque/1 -> Sum5/1
  Sum4/1 -> Gain3/1  "speed"
  Gain/1 -> Subsystem/1(p_int)
  Gain3/1 -> Subsystem/2(v_int)
  Gain4/1 -> Subsystem/3(kp_int)
  Gain5/1 -> Subsystem/4(kd_int)
  Gain6/1 -> Subsystem/5(t_int)
  Subsystem/1(Out2) -> Vector Concatenate/1
  Subsystem/2(Out1) -> Vector Concatenate/2
  Subsystem/4(Out4) -> Vector Concatenate/4
  Subsystem/5(Out5) -> Vector Concatenate/5
  Subsystem/6(Out6) -> Vector Concatenate/6
  Subsystem/7(Out7) -> Vector Concatenate/7
  Subsystem/3(Out3) -> Vector Concatenate/3
  Subsystem/8(Out8) -> Vector Concatenate/8

== system new_control/Subsystem3/Left Motor Velocity/Subsystem/Subsystem2 ==
  Enable : Inport
  Velocity : Inport  Port=2
  Mux1 : Mux  Inputs=5
  Subsystem : Subsystem
  Subsystem2 : Subsystem
  Enter_motor_mode : Outport
  Velocity_value : Outport  Port=2
  wires:
  Subsystem2/3(Out3) -> Mux1/3
  Subsystem2/2(Out2) -> Mux1/2
  Subsystem2/4(Out4) -> Mux1/4
  Subsystem2/1(Out1) -> Mux1/1
  Subsystem/1(Out1) -> Velocity_value/1
  Mux1/1 -> Enter_motor_mode/1
  Enable/1 -> Mux1/5
  Velocity/1 -> Subsystem/1(In1)

== system new_control/Subsystem3/Right Motor Velocity/Motor Actual Position Receive/CHINESE CORRECTION ==
  position : Inport
  Enable : EnablePort  StatesWhenEnabling=reset
  Abs : Abs  SaturateOnIntegerOverflow=off
  Constant2 : Constant
  Constant3 : Constant  Value=0
  Memory : Memory
  Subsystem : Subsystem
  Sum : Sum  Inputs=|+-
  Sum1 : Sum  Inputs=+-
  Switch1 : Switch  Criteria=u2 > Threshold  Threshold=20  SaturateOnIntegerOverflow=off  InputSameDT=off
  Out1 : Outport
  wires:
  Constant2/1 -> Switch1/1
  position/1 -> Sum1/1, Sum/1, Memory/1
  Sum/1 -> Abs/1, Subsystem/1(In1)
  Sum1/1 -> Out1/1
  Abs/1 -> Switch1/2
  Constant3/1 -> Switch1/3
  Switch1/1 -> Subsystem/Enable
  Memory/1 -> Sum/2
  Subsystem/1(Out1) -> Sum1/2

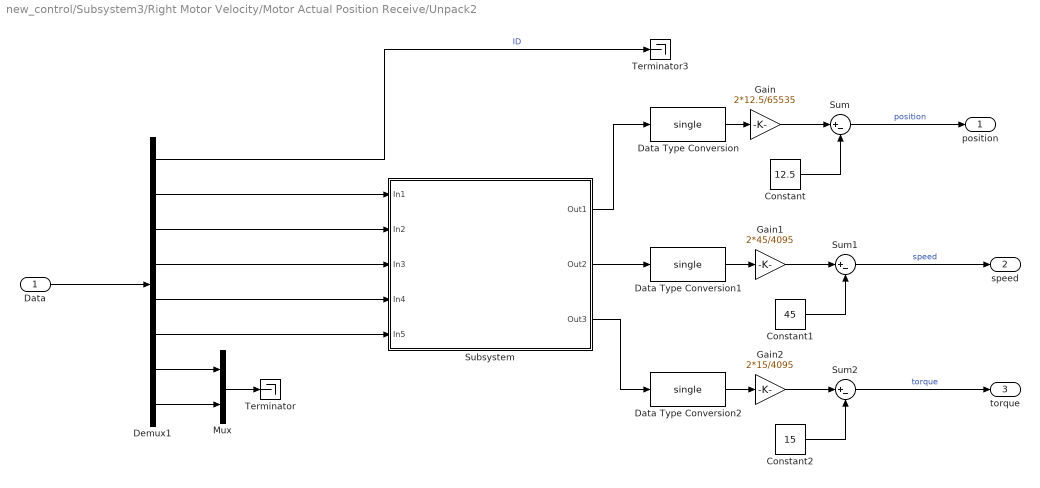
== system new_control/Subsystem3/Right Motor Velocity/Motor Actual Position Receive/Unpack2 ==
  Data : Inport
  Constant : Constant  Value=12.5
  Constant1 : Constant  Value=45
  Constant2 : Constant  Value=15
  Data Type Conversion : DataTypeConversion  OutDataTypeStr=single  SaturateOnIntegerOverflow=off  RndMeth=Floor
  Data Type Conversion1 : DataTypeConversion  OutDataTypeStr=single  SaturateOnIntegerOverflow=off  RndMeth=Floor
  Data Type Conversion2 : DataTypeConversion  OutDataTypeStr=single  SaturateOnIntegerOverflow=off  RndMeth=Floor
  Demux1 : Demux  Outputs=8
  Gain : Gain  Gain=2*12.5/65535  RndMeth=Round
  Gain1 : Gain  Gain=2*45/4095  RndMeth=Round
  Gain2 : Gain  Gain=2*15/4095  RndMeth=Round
  Mux : Mux  Inputs=2
  Subsystem : Subsystem
  Sum : Sum  Inputs=|+-
  Sum1 : Sum  Inputs=|+-
  Sum2 : Sum  Inputs=|+-
  Terminator : Terminator
  Terminator3 : Terminator
  position : Outport
  speed : Outport  Port=2
  torque : Outport  Port=3
  wires:
  Demux1/1 -> Terminator3/1  "ID"
  Demux1/7 -> Mux/1
  Demux1/8 -> Mux/2
  Demux1/2 -> Subsystem/1(In1)
  Demux1/3 -> Subsystem/2(In2)
  Demux1/4 -> Subsystem/3(In3)
  Demux1/5 -> Subsystem/4(In4)
  Demux1/6 -> Subsystem/5(In5)
  Subsystem/1(Out1) -> Data Type Conversion/1
  Gain/1 -> Sum/1
  Constant/1 -> Sum/2
  Data Type Conversion/1 -> Gain/1
  Gain1/1 -> Sum1/1
  Data Type Conversion1/1 -> Gain1/1
  Constant1/1 -> Sum1/2
  Gain2/1 -> Sum2/1
  Data Type Conversion2/1 -> Gain2/1
  Constant2/1 -> Sum2/2
  Subsystem/2(Out2) -> Data Type Conversion1/1
  Subsystem/3(Out3) -> Data Type Conversion2/1
  Sum2/1 -> torque/1  "torque"
  Mux/1 -> Terminator/1
  Data/1 -> Demux1/1
  Sum/1 -> position/1  "position"
  Sum1/1 -> speed/1  "speed"

== system new_control/Subsystem3/Right Motor Velocity/Subsystem/CAN Pack1 ==
  Position : Inport
  Velocity : Inport  Port=2
  Kp : Inport  Port=3
  Kd : Inport  Port=4
  Torque : Inport  Port=5
  Constant3 : Constant  Value=-12.5  OutDataTypeStr=single
  Constant4 : Constant  Value=-45  OutDataTypeStr=single
  Constant5 : Constant  Value=-15  OutDataTypeStr=single
  Gain : Gain  Gain=65535/(2*12.5)  OutDataTypeStr=uint16  RndMeth=Round
  Gain3 : Gain  Gain=4095/(2*45)  OutDataTypeStr=fixdt(0,12,0)  RndMeth=Round
  Gain4 : Gain  Gain=4095/500  OutDataTypeStr=fixdt(0,12,0)  RndMeth=Round
  Gain5 : Gain  Gain=4095/5  OutDataTypeStr=fixdt(0,12,0)  RndMeth=Round
  Gain6 : Gain  Gain=4095/(2*15)  OutDataTypeStr=fixdt(0,12,0)  RndMeth=Round
  Subsystem : Subsystem
  Sum3 : Sum  Inputs=|+-
  Sum4 : Sum  Inputs=|+-
  Sum5 : Sum  Inputs=|+-
  Vector Concatenate : Concatenate  NumInputs=8
  CAN Data : Outport
  wires:
  Velocity/1 -> Sum4/1
  Kp/1 -> Gain4/1
  Kd/1 -> Gain5/1
  Vector Concatenate/1 -> CAN Data/1
  Constant3/1 -> Sum3/2
  Sum3/1 -> Gain/1  "position"
  Position/1 -> Sum3/1
  Constant4/1 -> Sum4/2
  Constant5/1 -> Sum5/2
  Sum5/1 -> Gain6/1  "torque"
  Torque/1 -> Sum5/1
  Sum4/1 -> Gain3/1  "speed"
  Gain/1 -> Subsystem/1(p_int)
  Gain3/1 -> Subsystem/2(v_int)
  Gain4/1 -> Subsystem/3(kp_int)
  Gain5/1 -> Subsystem/4(kd_int)
  Gain6/1 -> Subsystem/5(t_int)
  Subsystem/1(Out2) -> Vector Concatenate/1
  Subsystem/2(Out1) -> Vector Concatenate/2
  Subsystem/4(Out4) -> Vector Concatenate/4
  Subsystem/5(Out5) -> Vector Concatenate/5
  Subsystem/6(Out6) -> Vector Concatenate/6
  Subsystem/7(Out7) -> Vector Concatenate/7
  Subsystem/3(Out3) -> Vector Concatenate/3
  Subsystem/8(Out8) -> Vector Concatenate/8

== system new_control/Subsystem3/Right Motor Velocity/Subsystem/Subsystem2 ==
  Enable : Inport
  Velocity : Inport  Port=2
  Mux1 : Mux  Inputs=5
  Subsystem : Subsystem
  Subsystem2 : Subsystem
  Enter_motor_mode : Outport
  Velocity_value : Outport  Port=2
  wires:
  Subsystem2/3(Out3) -> Mux1/3
  Subsystem2/2(Out2) -> Mux1/2
  Subsystem2/4(Out4) -> Mux1/4
  Subsystem2/1(Out1) -> Mux1/1
  Subsystem/1(Out1) -> Velocity_value/1
  Mux1/1 -> Enter_motor_mode/1
  Enable/1 -> Mux1/5
  Velocity/1 -> Subsystem/1(In1)

== system new_control/Subsystem1/Left Motor Velocity1/Motor Actual Position Receive/CHINESE CORRECTION/Subsystem ==
  In1 : Inport
  Enable : EnablePort
  Memory : Memory
  Sum : Sum  Inputs=|++
  Out1 : Outport
  wires:
  In1/1 -> Sum/1
  Sum/1 -> Out1/1, Memory/1
  Memory/1 -> Sum/2

== system new_control/Subsystem1/Left Motor Velocity1/Motor Actual Position Receive/Unpack2/Subsystem ==
  In1 : Inport
  In2 : Inport  Port=2
  In3 : Inport  Port=3
  In4 : Inport  Port=4
  In5 : Inport  Port=5
  Bitwise AND : simulink/Logic and Bit Operations/Bitwise Operator  logicop=AND  UseBitMask=on  BitMask=bin2dec('0000000000001111')  BitMaskRealWorld=Stored Integer
  Bitwise OR : simulink/Logic and Bit Operations/Bitwise Operator  logicop=OR  UseBitMask=off  NumInputPorts=2  BitMask=bin2dec('11011001')  BitMaskRealWorld=Stored Integer
  Bitwise OR1 : simulink/Logic and Bit Operations/Bitwise Operator  logicop=OR  UseBitMask=off  NumInputPorts=2  BitMask=bin2dec('11011001')  BitMaskRealWorld=Stored Integer
  Bitwise OR2 : simulink/Logic and Bit Operations/Bitwise Operator  logicop=OR  UseBitMask=off  NumInputPorts=2  BitMask=bin2dec('11011001')  BitMaskRealWorld=Stored Integer
  Constant : Constant  Value=8  OutDataTypeStr=uint16
  Constant1 : Constant  Value=4  OutDataTypeStr=uint16
  Constant2 : Constant  Value=4  OutDataTypeStr=uint16
  Constant4 : Constant  Value=8  OutDataTypeStr=uint16
  Shift Arithmetic1 : ArithShift  BitShiftNumberSource=Input port  BitShiftNumber=8  BitShiftDirection=Left
  Shift Arithmetic2 : ArithShift  BitShiftNumberSource=Input port  BitShiftNumber=8  BitShiftDirection=Left
  Shift Arithmetic3 : ArithShift  BitShiftNumberSource=Input port  BitShiftNumber=8  BitShiftDirection=Right
  Shift Arithmetic4 : ArithShift  BitShiftNumberSource=Input port  BitShiftNumber=8  BitShiftDirection=Left
  Out1 : Outport
  Out2 : Outport  Port=2
  Out3 : Outport  Port=3
  wires:
  Bitwise AND/1 -> Shift Arithmetic4/1
  In5/1 -> Bitwise OR2/1
  Shift Arithmetic1/1 -> Bitwise OR1/1
  In1/1 -> Shift Arithmetic1/1
  Shift Arithmetic2/1 -> Bitwise OR/1
  Shift Arithmetic3/1 -> Bitwise OR/2
  Shift Arithmetic4/1 -> Bitwise OR2/2
  In2/1 -> Bitwise OR1/2
  Bitwise OR1/1 -> Out1/1
  Bitwise OR2/1 -> Out3/1
  In3/1 -> Shift Arithmetic2/1
  Constant4/1 -> Shift Arithmetic4/2
  Constant2/1 -> Shift Arithmetic3/2
  Constant1/1 -> Shift Arithmetic2/2
  Constant/1 -> Shift Arithmetic1/2
  Bitwise OR/1 -> Out2/1
  In4/1 -> Shift Arithmetic3/1, Bitwise AND/1

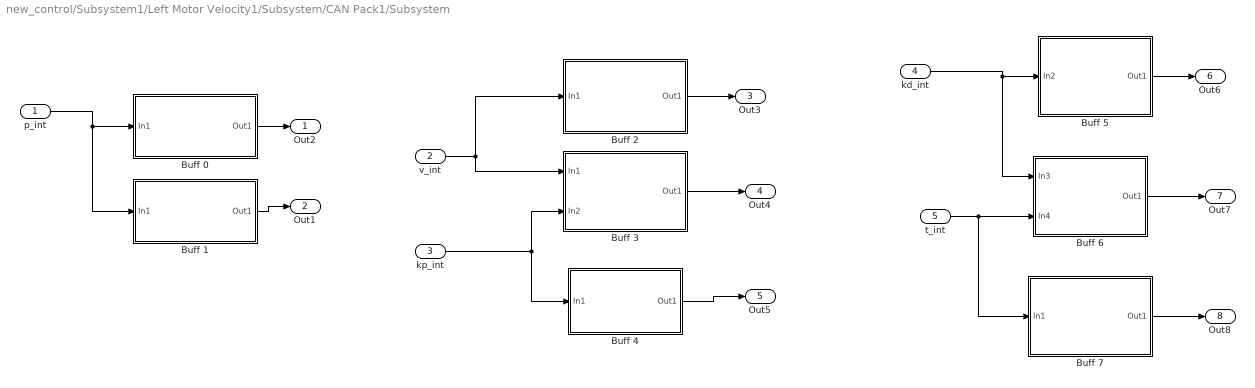
== system new_control/Subsystem1/Left Motor Velocity1/Subsystem/CAN Pack1/Subsystem ==
  p_int : Inport
  v_int : Inport  Port=2
  kp_int : Inport  Port=3
  kd_int : Inport  Port=4
  t_int : Inport  Port=5
  Buff 0 : Subsystem
  Buff 1 : Subsystem
  Buff 2 : Subsystem
  Buff 3 : Subsystem
  Buff 4 : Subsystem
  Buff 5 : Subsystem
  Buff 6 : Subsystem
  Buff 7 : Subsystem
  Out2 : Outport
  Out1 : Outport  Port=2
  Out3 : Outport  Port=3
  Out4 : Outport  Port=4
  Out5 : Outport  Port=5
  Out6 : Outport  Port=6
  Out7 : Outport  Port=7
  Out8 : Outport  Port=8
  wires:
  Buff 5/1(Out1) -> Out6/1
  Buff 7/1(Out1) -> Out8/1
  Buff 6/1(Out1) -> Out7/1
  Buff 0/1(Out1) -> Out2/1
  Buff 1/1(Out1) -> Out1/1
  Buff 2/1(Out1) -> Out3/1
  Buff 4/1(Out1) -> Out5/1
  Buff 3/1(Out1) -> Out4/1
  p_int/1 -> Buff 0/1(In1), Buff 1/1(In1)
  v_int/1 -> Buff 3/1(In1), Buff 2/1(In1)
  kd_int/1 -> Buff 6/1(In3), Buff 5/1(In2)
  kp_int/1 -> Buff 3/2(In2), Buff 4/1(In1)
  t_int/1 -> Buff 7/1(In1), Buff 6/2(In4)
